simulink model "EngSpd_DD"  (R2016b)
settings: configuration reference "CodeGenConfigSet" (kept outside this file)
values from neighbouring files (symbols this model uses):
  EngSpd_rPs_C = Calibration.Parameter    [init_EngSpd_DD.m]    (also in init_EngSpd_DD_SIL.m = Simulink.Parameter)
  EpmSpd_numPlsPerRot_C = Calibration.Parameter    [init_EngSpd_DD.m]    (also in init_EngSpd_DD_SIL.m = Simulink.Parameter)
settings Model: Creator=Wei Liang  LastModifiedBy=yangyang
settings ConfigSetRef: SourceLocation=Base Workspace

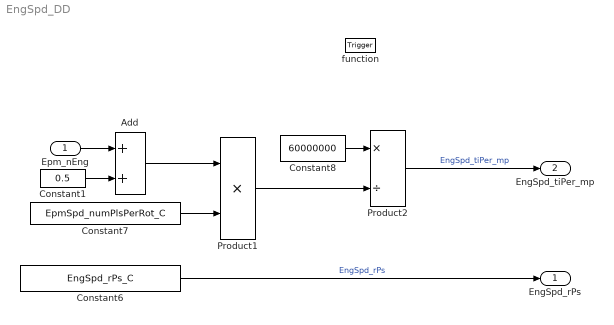
== system EngSpd_DD ==
  Epm_nEng : Inport  Tag=rpm  Description=Engine speed  OutMin=0  OutMax=6000  OutDataTypeStr=EngSpeed_rpm
  function : TriggerPort  TriggerType=function-call  VariantControl=Variant
  Add : Sum  SaturateOnIntegerOverflow=on  InputSameDT=on
  Constant1 : Constant  Value=0.5  OutDataTypeStr=Inherit: Inherit via back propagation
  Constant6 : Constant  Value=EngSpd_rPs_C  SampleTime=-1
  Constant7 : Constant  Value=EpmSpd_numPlsPerRot_C
  Constant8 : Constant  Value=60000000  OutDataTypeStr=uint32
  Product1 : Product  RndMeth=Round  SaturateOnIntegerOverflow=on
  Product2 : Product  Inputs=*/  OutDataTypeStr=Inherit: Inherit via back propagation  RndMeth=Round  SaturateOnIntegerOverflow=on
  EngSpd_rPs : Outport  Tag=%  Description=Structure containing parameters for PWM output power stage error handling for engine speed PWM out  OutMin=0  OutMax=100  OutDataTypeStr=DutyCycle_rate
  EngSpd_tiPer_mp : Outport  Tag=us  Description=signal period duration  Port=2  OutMin=-107374182  OutMax=107374182  OutDataTypeStr=Time_PwmHigh_us
  wires:
  Constant7/1 -> Product1/2
  Constant8/1 -> Product2/1
  Product1/1 -> Product2/2
  Product2/1 -> EngSpd_tiPer_mp/1  "EngSpd_tiPer_mp"
  Constant6/1 -> EngSpd_rPs/1  "EngSpd_rPs"
  Add/1 -> Product1/1
  Constant1/1 -> Add/2
  Epm_nEng/1 -> Add/1
